simulink model "T5_Output_Feedback_LinearMPC"  (R2023a)
settings: Solver=ode4  StartTime=0.0  StopTime=inf  FixedStep=0.1  RelTol=1e-3
model workspace (MAT data in the model file):
  aa = 1
values from neighbouring files (symbols this model uses):
  A = ds.a    [Linear_MPC.m]
  Ac = [0,0,1,0 ... (first row only)    [Linerized_Parameters.m]
  B = ds.b    [Linear_MPC.m]
  B_p = 0.01    [Heli_Parameters.m]
  B_y = 0.08    [Heli_Parameters.m]
  Bc = [0,0 ... (first row only)    [Linerized_Parameters.m]
  C = ds.c    [Linear_MPC.m]
  Cc = [1,0,0,0 ... (first row only)    [Linerized_Parameters.m]
  g = 9.81    [Heli_Parameters.m]
  J_eqp = 0.0172    [Heli_Parameters.m]
  J_eqy = 0.0210    (= 0.021)    [Heli_Parameters.m]
  K_pp = 0.0556    [Heli_Parameters.m]
  K_py = 0.005    [Heli_Parameters.m]
  K_yp = 0.15    [Heli_Parameters.m]
  K_yy = 0.21084    [Heli_Parameters.m]
  l_cm = 0.015    [Heli_Parameters.m]
  m_heli = 0.479    [Heli_Parameters.m]
  N = 20    [Linear_MPC.m]
  nu = size(B,2)    [Linear_MPC.m]
  nx = size(A,1)    [Linear_MPC.m]
  ny = size(C,1)    [Linear_MPC.m]
  nz = N*(nx + nu + 2*ny)    [Linear_MPC.m]
  p_op = pi/2    (= 1.57079632679)    [Linerized_Parameters.m]
  t_op = (-10*pi)/180    (= -0.174532925199)    [Linerized_Parameters.m]
  V_mp_op = (K_yy* m_heli*g*cos(t_op)*l_cm  )/((K_yy*K_pp-K_yp*K_py))    [Linerized_Parameters.m]
  V_my_op = (K_yp* V_mp_op)/K_yy    [Linerized_Parameters.m]
  zL = (-Inf*ones(nz,1))    [Linear_MPC.m]
  zU = (Inf*ones(nz,1))    [Linear_MPC.m]
undefined symbols (not defined in the file or in its folder): L
libraries: realtime_pacer_lib x1
settings Model: Creator=aleho  LastModifiedBy=aleho

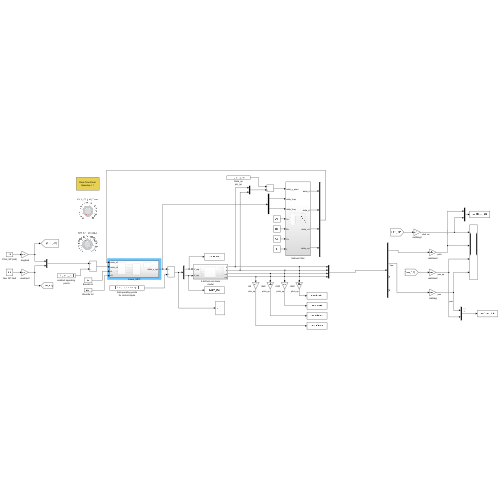
[thumbnail: Simulink's stored preview of the top-level diagram]
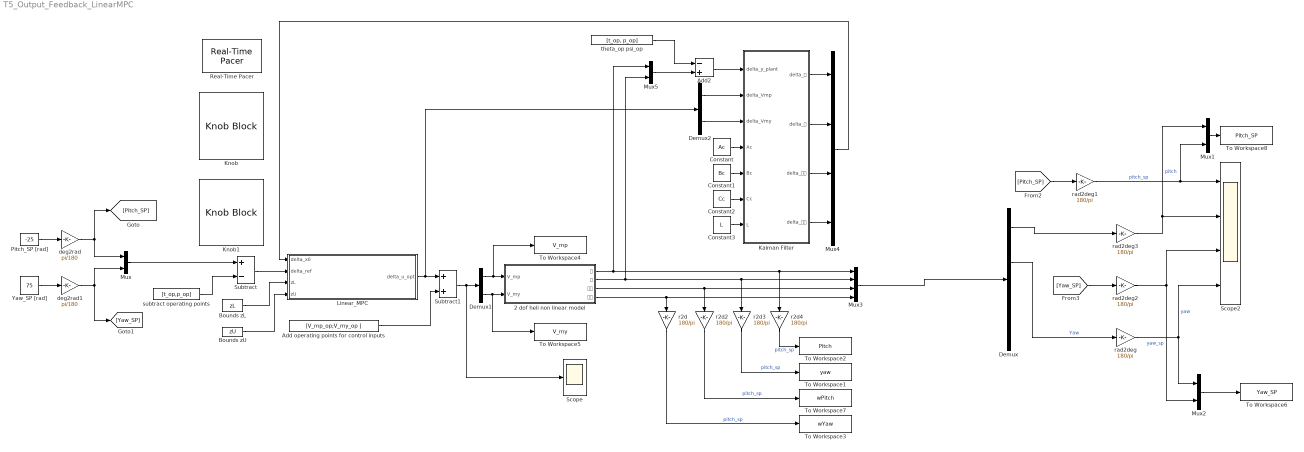
== system T5_Output_Feedback_LinearMPC ==
  2 dof heli non linear model : Subsystem
  Add operating points for control inputs : Constant  Value=[V_mp_op;V_my_op ]
  Add2 : Sum  Inputs=-+
  Bounds zL : Constant  Value=zL
  Bounds zU : Constant  Value=zU
  Constant : Constant  Value=Ac
  Constant1 : Constant  Value=Bc
  Constant2 : Constant  Value=Cc
  Constant3 : Constant  Value=L
  Demux : Demux
  Demux1 : Demux  Outputs=2
  Demux2 : Demux  Outputs=2
  Kalman Filter : Subsystem
  Knob : KnobBlock  ScaleMin=-20  ScaleMax=45  TickInterval=4
  Knob1 : KnobBlock  ScaleMax=180  TickInterval=10
  Linear_MPC : Subsystem
  Mux{,1..2,5} (4 alike) : Mux  Inputs=2
  Mux3 : Mux
  Mux4 : Mux
  Pitch_SP [rad] : Constant  Value=-25
  Real-Time Pacer : realtime_pacer_lib/Real-Time Pacer  simTimePerRealTime=1
  Scope : Scope
  Scope2 : Scope  NumInputPorts=4
  Subtract : Sum  Inputs=+-
  Subtract1 : Sum
  To Workspace1 : ToWorkspace  VariableName=yaw  SaveFormat=Timeseries  SampleTime=-1
  To Workspace2 : ToWorkspace  VariableName=Pitch  SaveFormat=Timeseries  SampleTime=-1
  To Workspace3 : ToWorkspace  VariableName=wYaw  SaveFormat=Timeseries  SampleTime=-1
  To Workspace4 : ToWorkspace  VariableName=V_mp  SaveFormat=Timeseries  SampleTime=-1
  To Workspace5 : ToWorkspace  VariableName=V_my  SaveFormat=Timeseries  SampleTime=-1
  To Workspace6 : ToWorkspace  VariableName=Yaw_SP  SaveFormat=Timeseries  SampleTime=-1
  To Workspace7 : ToWorkspace  VariableName=wPitch  SaveFormat=Timeseries  SampleTime=-1
  To Workspace8 : ToWorkspace  VariableName=Pitch_SP  SaveFormat=Timeseries  SampleTime=-1
  Yaw_SP [rad] : Constant  Value=75
  deg2rad : Gain  Gain=pi/180
  deg2rad1 : Gain  Gain=pi/180
  r2d{,2..4} (4 alike) : Gain  Gain=180/pi
  rad2deg{,1..3} (4 alike) : Gain  Gain=180/pi
  subtract operating points : Constant  Value=[t_op,p_op]
  theta_op psi_op : Constant  Value=[t_op, p_op]
  wires:
  Pitch_SP [rad]/1 -> deg2rad/1
  Yaw_SP [rad]/1 -> deg2rad1/1
  Subtract/1 -> Linear_MPC/2(delta_ref)
  Demux/1 -> rad2deg3/1
  Demux/2 -> rad2deg/1  "Yaw"
  Linear_MPC/1(delta_u_opt) -> Demux2/1, Subtract1/1
  Add operating points for control inputs/1 -> Subtract1/2
  Subtract1/1 -> Scope/1, Demux1/1
  Mux/1 -> Subtract/1
  subtract operating points/1 -> Subtract/2
  Demux1/1 -> To Workspace4/1, 2 dof heli non linear model/1(V_mp)
  Demux1/2 -> To Workspace5/1, 2 dof heli non linear model/2(V_my)
  2 dof heli non linear model/1(𝜃) -> r2d4/1, Mux3/1, Mux5/1
  2 dof heli non linear model/2(𝜓) -> r2d3/1, Mux3/2, Mux5/2
  2 dof heli non linear model/3(𝜔𝜃) -> r2d2/1, Mux3/3
  2 dof heli non linear model/4(𝜔𝜓) -> r2d/1, Mux3/4
  Mux3/1 -> Demux/1
  [Yaw_SP] -> rad2deg2/1
  rad2deg/1 -> Mux2/1, Scope2/4  "yaw"
  rad2deg3/1 -> Mux1/1, Scope2/2  "pitch"
  [Pitch_SP] -> rad2deg1/1
  deg2rad/1 -> Mux/1, [Pitch_SP]
  deg2rad1/1 -> [Yaw_SP], Mux/2
  rad2deg1/1 -> Mux1/2, Scope2/1  "pitch_sp"
  rad2deg2/1 -> Mux2/2, Scope2/3  "yaw_sp"
  Bounds zU/1 -> Linear_MPC/4(zU)
  Bounds zL/1 -> Linear_MPC/3(zL)
  Kalman Filter/1(delta_𝜃) -> Mux4/1
  Kalman Filter/2(delta_𝜓) -> Mux4/2
  Kalman Filter/3(delta_𝜔𝜃) -> Mux4/3
  Kalman Filter/4(delta_𝜔𝜓) -> Mux4/4
  Mux4/1 -> Linear_MPC/1(delta_x0)
  Constant/1 -> Kalman Filter/4(Ac)
  Constant1/1 -> Kalman Filter/5(Bc)
  Constant2/1 -> Kalman Filter/6(Cc)
  Constant3/1 -> Kalman Filter/7(L)
  Mux5/1 -> Add2/2
  Add2/1 -> Kalman Filter/1(delta_y_plant)
  theta_op psi_op/1 -> Add2/1
  Demux2/1 -> Kalman Filter/2(delta_Vmp)
  Demux2/2 -> Kalman Filter/3(delta_Vmy)
  Mux1/1 -> To Workspace8/1
  Mux2/1 -> To Workspace6/1
  r2d4/1 -> To Workspace2/1  "pitch_sp"
  r2d3/1 -> To Workspace1/1  "pitch_sp"
  r2d2/1 -> To Workspace7/1  "pitch_sp"
  r2d/1 -> To Workspace3/1  "pitch_sp"

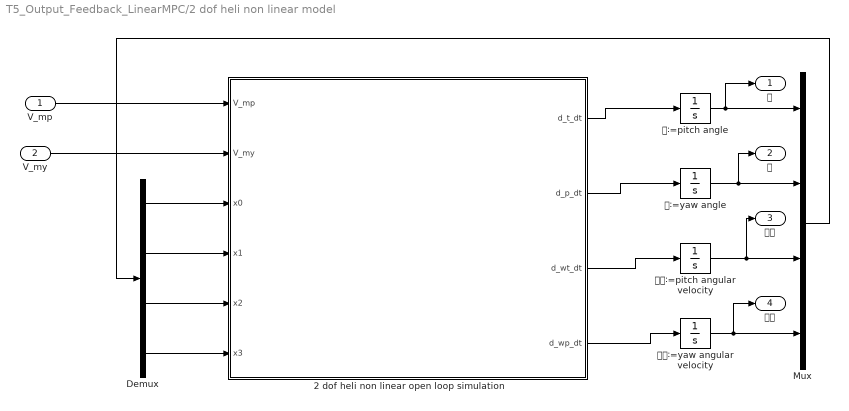
== system T5_Output_Feedback_LinearMPC/2 dof heli non linear model ==
  V_mp : Inport
  V_my : Inport  Port=2
  2 dof heli non linear open loop simulation : MATLAB Function  TreatAsAtomicUnit=on
  Demux : Demux
  Mux : Mux
  𝜃∶=pitch angle : Integrator  InitialCondition=-45*pi/180  LimitOutput=on  UpperSaturationLimit=pi/4  LowerSaturationLimit=-pi/4
  𝜓∶=yaw angle : Integrator  InitialCondition=pi/2  LimitOutput=on  UpperSaturationLimit=pi  LowerSaturationLimit=0
  𝜔𝜃∶=pitch angular velocity : Integrator
  𝜔𝜓∶=yaw angular velocity : Integrator
  𝜃 : Outport
  𝜓 : Outport  Port=2
  𝜔𝜃 : Outport  Port=3
  𝜔𝜓 : Outport  Port=4
  wires:
  V_mp/1 -> 2 dof heli non linear open loop simulation/1(V_mp)
  𝜔𝜃∶=pitch angular velocity/1 -> 𝜔𝜃/1, Mux/3
  Demux/4 -> 2 dof heli non linear open loop simulation/6(x3)
  𝜔𝜓∶=yaw angular velocity/1 -> 𝜔𝜓/1, Mux/4
  Mux/1 -> Demux/1
  𝜃∶=pitch angle/1 -> 𝜃/1, Mux/1
  𝜓∶=yaw angle/1 -> 𝜓/1, Mux/2
  2 dof heli non linear open loop simulation/1(d_t_dt) -> 𝜃∶=pitch angle/1
  V_my/1 -> 2 dof heli non linear open loop simulation/2(V_my)
  Demux/1 -> 2 dof heli non linear open loop simulation/3(x0)
  Demux/3 -> 2 dof heli non linear open loop simulation/5(x2)
  Demux/2 -> 2 dof heli non linear open loop simulation/4(x1)
  2 dof heli non linear open loop simulation/2(d_p_dt) -> 𝜓∶=yaw angle/1
  2 dof heli non linear open loop simulation/4(d_wp_dt) -> 𝜔𝜓∶=yaw angular velocity/1
  2 dof heli non linear open loop simulation/3(d_wt_dt) -> 𝜔𝜃∶=pitch angular velocity/1

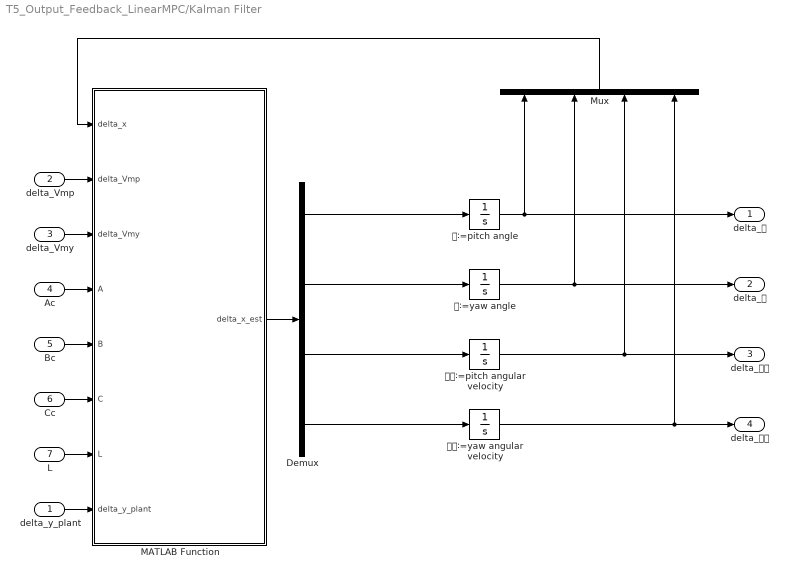
== system T5_Output_Feedback_LinearMPC/Kalman Filter ==
  delta_y_plant : Inport
  delta_Vmp : Inport  Port=2
  delta_Vmy : Inport  Port=3
  Ac : Inport  Port=4
  Bc : Inport  Port=5
  Cc : Inport  Port=6
  L : Inport  Port=7
  Demux : Demux
  MATLAB Function : MATLAB Function  TreatAsAtomicUnit=on
  Mux : Mux
  𝜃∶=pitch angle : Integrator  InitialCondition=-45*pi/180  LimitOutput=on  UpperSaturationLimit=45*pi/180-t_op  LowerSaturationLimit=(-45*pi/180)+t_op
  𝜓∶=yaw angle : Integrator  InitialCondition=pi/2  LimitOutput=on  UpperSaturationLimit=pi-p_op  LowerSaturationLimit=0-p_op
  𝜔𝜃∶=pitch angular velocity : Integrator  LimitOutput=on  UpperSaturationLimit=2  LowerSaturationLimit=-2
  𝜔𝜓∶=yaw angular velocity : Integrator  LimitOutput=on  UpperSaturationLimit=2  LowerSaturationLimit=-2
  delta_𝜃 : Outport
  delta_𝜓 : Outport  Port=2
  delta_𝜔𝜃 : Outport  Port=3
  delta_𝜔𝜓 : Outport  Port=4
  wires:
  delta_Vmp/1 -> MATLAB Function/2(delta_Vmp)
  delta_Vmy/1 -> MATLAB Function/3(delta_Vmy)
  MATLAB Function/1(delta_x_est) -> Demux/1
  Demux/1 -> 𝜃∶=pitch angle/1
  Demux/2 -> 𝜓∶=yaw angle/1
  Demux/3 -> 𝜔𝜃∶=pitch angular velocity/1
  Demux/4 -> 𝜔𝜓∶=yaw angular velocity/1
  𝜔𝜓∶=yaw angular velocity/1 -> Mux/4, delta_𝜔𝜓/1
  𝜔𝜃∶=pitch angular velocity/1 -> Mux/3, delta_𝜔𝜃/1
  𝜃∶=pitch angle/1 -> Mux/1, delta_𝜃/1
  𝜓∶=yaw angle/1 -> Mux/2, delta_𝜓/1
  Mux/1 -> MATLAB Function/1(delta_x)
  Ac/1 -> MATLAB Function/4(A)
  Bc/1 -> MATLAB Function/5(B)
  Cc/1 -> MATLAB Function/6(C)
  L/1 -> MATLAB Function/7(L)
  delta_y_plant/1 -> MATLAB Function/8(delta_y_plant)

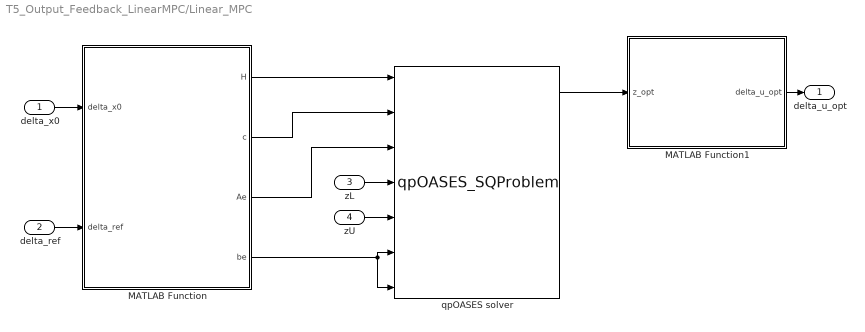
== system T5_Output_Feedback_LinearMPC/Linear_MPC ==
  delta_x0 : Inport
  delta_ref : Inport  Port=2
  zL : Inport  Port=3
  zU : Inport  Port=4
  MATLAB Function : MATLAB Function  TreatAsAtomicUnit=on
  MATLAB Function1 : MATLAB Function  TreatAsAtomicUnit=on
  qpOASES solver : S-Function  FunctionName=qpOASES_SQProblem  SFunctionDeploymentMode=off  EnableBusSupport=off
  delta_u_opt : Outport
  wires:
  MATLAB Function/3(Ae) -> qpOASES solver/3
  delta_x0/1 -> MATLAB Function/1(delta_x0)
  MATLAB Function/4(be) -> qpOASES solver/7, qpOASES solver/6
  MATLAB Function/2(c) -> qpOASES solver/2
  MATLAB Function1/1(delta_u_opt) -> delta_u_opt/1
  delta_ref/1 -> MATLAB Function/2(delta_ref)
  qpOASES solver/1 -> MATLAB Function1/1(z_opt)
  MATLAB Function/1(H) -> qpOASES solver/1
  zL/1 -> qpOASES solver/4
  zU/1 -> qpOASES solver/5

== matlab function T5_Output_Feedback_LinearMPC/Linear_MPC/MATLAB Function1 ==
  data: z_opt input; delta_u_opt output
function delta_u_opt = select_first_control_move(z_opt)
delta_u_opt = z_opt(1:2);

== matlab function T5_Output_Feedback_LinearMPC/Linear_MPC/MATLAB Function ==
  data: delta_x0 input size=[4 1]; H output; delta_ref input; c output; Ae output; be output; A parameter; B parameter; C parameter; N parameter; nz parameter; ny parameter; nx parameter; nu parameter
function [H,c,Ae,be] = QP_formulation(delta_x0,delta_ref,A, B, C, N, nz, ny, nx, nu)

del_x0 = delta_x0; %States

%References/Setpoints
delta_ref_N = [ones(1,N).*delta_ref(1);
                ones(1,N).*delta_ref(2)];

Q=diag([3.0 3.0]);  %tuning weight of error
P= diag([1 1]);     %tuning weight of inputs

H11 = kron(eye(N),P);
H22 = zeros(N*nx,N*nx);
H33 = kron(eye(N),Q);
H44 = zeros(N*ny,N*ny);
H_mat = blkdiag(H11,H22,H33,H44);

H = H_mat(:);
c = zeros(nz,1);

%First constraint
Ae1u = -kron(eye(N),B);
Ae1x = eye(N*nx)-kron(diag(ones(N-abs(-1),1),-1),A);
Ae1e = zeros(N*nx,N*ny);
Ae1y = zeros(N*nx,N*ny);
be1 = [A*del_x0;zeros((N-1)*nx,1)];

%Second constraint
Ae2u = zeros(N*ny,N*nu);
Ae2x = -kron(eye(N),C);
Ae2e = zeros(N*ny,N*ny);
Ae2y = eye(N*ny);
be2 = zeros(N*ny,1);

%Third constraint
Ae3u = zeros(N*ny,N*nu);
Ae3x = zeros(N*ny,N*nx);
Ae3e = eye(N*ny);
Ae3y = eye(N*ny);
be3 = reshape(delta_ref_N,N*ny,1);

Ae_mat=[Ae1u Ae1x Ae1e Ae1y;
        Ae2u Ae2x Ae2e Ae2y;
        Ae3u Ae3x Ae3e Ae3y];

Ae = Ae_mat(:);
be=[be1;be2;be3];

== matlab function T5_Output_Feedback_LinearMPC/Kalman Filter/MATLAB Function ==
  data: delta_x input; delta_Vmp input; delta_Vmy input; A input; B input; C input; L input; delta_y_plant input; delta_x_est output
function delta_x_est  = linear_observer(delta_x, delta_Vmp, delta_Vmy, A,B,C,L, delta_y_plant)

y_est = C*delta_x;
delta_x_est = A*delta_x+B*[delta_Vmp;delta_Vmy] + L*(delta_y_plant-y_est); % L = Kf(Kalman gain)

%delta_x1_hat = delta_x(1);
%delta_x2_hat = delta_x(2);
%delta_x3_hat = delta_x(3);
%delta_x4_hat = delta_x(4);

== matlab function T5_Output_Feedback_LinearMPC/2 dof heli non linear model/2 dof heli non linear open loop simulation ==
  data: V_mp input; V_my input; d_t_dt output; d_p_dt output; d_wt_dt output; d_wp_dt output; x0 input; x1 input; x2 input; x3 input; l_cm parameter; m_heli parameter; J_eqp parameter; J_eqy parameter; g parameter; K_pp parameter; K_yy parameter; K_py parameter; K_yp parameter; B_p parameter; B_y parameter
function [d_t_dt,d_p_dt,d_wt_dt,d_wp_dt] =  heli_2_dof_ODE_eqs(V_mp,V_my,x0,x1,x2,x3,l_cm, m_heli, J_eqp, J_eqy, g, K_pp, K_yy, K_py, K_yp, B_p, B_y)
% States
t = x0;    % pitch angle ( theta )
p = x1;    % yaw angle ( psi )
wt = x2;   % pitch angular velocity ( Omega theta )
wp = x3;   % yaw angular velocity ( Omega psi )

% ODEs
% pitch angle
d_t_dt = wt;

% yaw angle
d_p_dt = wp;

% pitch angular velocity
d_wt_dt = ((K_pp*V_mp)/(J_eqp+m_heli*l_cm^2)) - ((K_py*V_my)/(J_eqp+m_heli*l_cm^2))...
    - ((B_p*wt+m_heli*wp^2*sin(t)*l_cm^2*cos(t)+m_heli*g*cos(t)*l_cm) / (J_eqp+m_heli*l_cm^2));

% yaw angular velocity
d_wp_dt = ((K_yp*V_mp)/(J_eqy+m_heli*cos(t)^2*l_cm^2)) -...
    ((K_yy*V_my)/(J_eqy+m_heli*cos(t)^2*l_cm^2)) +...
    ((2*m_heli*wp*sin(t)*l_cm^2*cos(t)*wt)/(J_eqy+m_heli*cos(t)^2*l_cm^2))...
    - ((B_y*wp)/(J_eqy+m_heli*cos(t)^2*l_cm^2));
